simulink model "MVC2026_sim"  (R2023b)
settings: Solver=ode23t  StartTime=0.0  StopTime=inf  FixedStep=Ts  RelTol=1e-3
values from neighbouring files (symbols this model uses):
  saveDataSampling = 0.01    [main.m]
undefined symbols (not defined in the file or in its folder): BAT, BUS, CH, CTRLpmsm, DiscIntNeverNeededParam, EMS, LoadRef, MOT, TraceRef, Ts, VEH, WindRef
libraries: nesl_utility x50, fl_lib x28, ee_lib x19, simulink x9, slpidlib x5, eeTransforms x4, sdl_lib x4, batteryecm_lib x1, eeGeneralControl x1
(part 1 of 3)
settings Model: SimulationMode=accelerator  Creator=ortolud16324  LastModifiedBy=ortolud16324
settings SolverCC: SolverResetMethod=Robust
settings DebuggingCC: SignalRangeChecking=warning

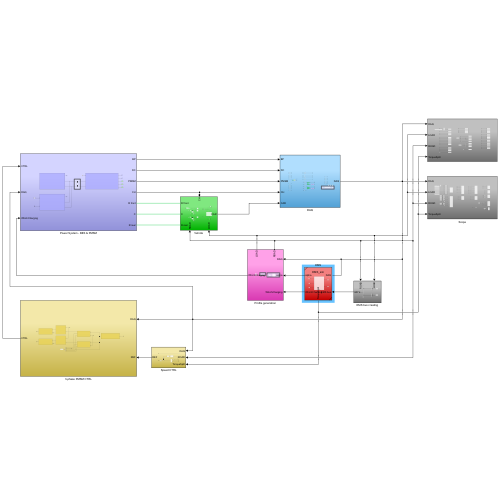
[thumbnail: Simulink's stored preview of the top-level diagram]
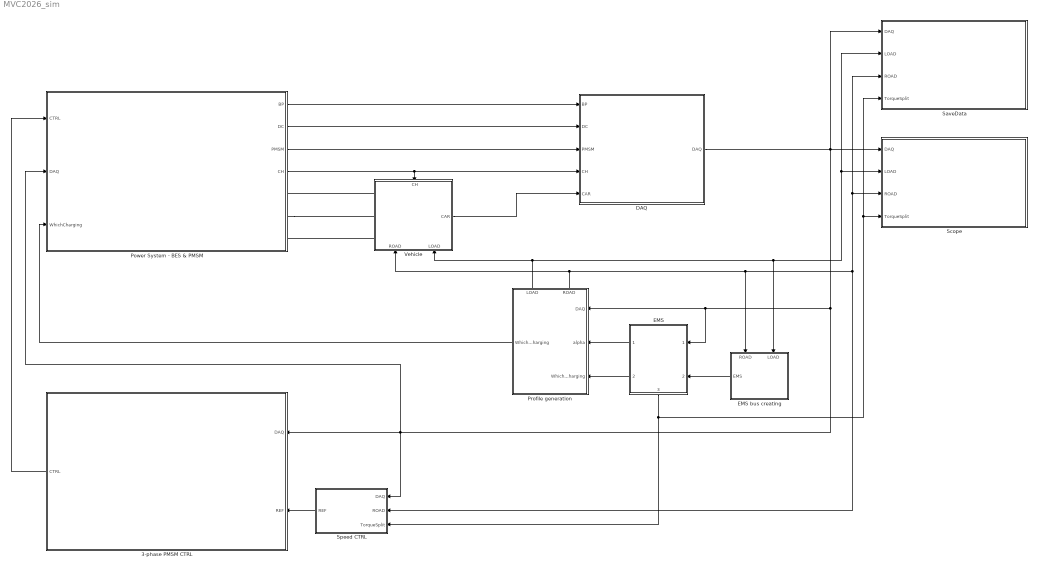
== system MVC2026_sim ==
  3-phase PMSM CTRL : Subsystem
  DAQ : Subsystem
  EMS : Subsystem  ReferencedSubsystem=EMS_sim
      settings: PortSchema="{\"entries\":[{\"content\":{\"sides\":[{\"content\":{\"connectorIds\":[\"In1\",\"In2\"]},\"type\":\"ConnectorPlacement.EquallySpacedRectSide\",\"uuid\":\"3854e963-bedd-46a1-9385-3ff6107fc6b9\"},{\"content\":{\"connectorIds\":[\"Out1\",\"Out2\"],\"side\":\"RIGHT\"},\"type\":\"ConnectorPlacement.EquallySpacedRectSide\",\"uuid\":\"f1426a81-f9cd-4ff1-8bf2-5f138fc7a080\"},{\"content\":{\"side\":\"TOP\"},\"type\":\"ConnectorPlacement.EquallySpacedRectSide\",\"uuid\":\"35da82e6-a4ef-4411-bef0-4d143ba62e69\"},{\"content\":{\"connectorIds\":[\"Out3\"],\"side\":\"BOTTOM\"},\"type\":\"ConnectorPlacement.EquallySpacedRectSide\",\"uuid\":\"49263484-0624-468a-bbdd-494b3d0a840d\"}]},\"type\":\"ConnectorPlacement.EquallySpacedConnector\",\"uuid\":\"bda56c1c-9437-4abe-9543-748b3b8cdce9\"}],\"packageUris\":[\"http://schema.mathworks.com/mf0/Connector/R2020b\"],\"version\":\"1.0\"}"
  EMS bus creating : Subsystem
      settings: PortSchema="{\"entries\":[{\"content\":{\"sides\":[{\"content\":{},\"type\":\"ConnectorPlacement.EquallySpacedRectSide\",\"uuid\":\"21c2c49d-f847-40d8-a3b7-36d147e58b7f\"},{\"content\":{\"connectorIds\":[\"Out1\"],\"side\":\"RIGHT\"},\"type\":\"ConnectorPlacement.EquallySpacedRectSide\",\"uuid\":\"241bf6a1-27e1-42c3-94c6-8bce09631f1d\"},{\"content\":{\"connectorIds\":[\"In1\",\"In2\"],\"side\":\"TOP\"},\"type\":\"ConnectorPlacement.EquallySpacedRectSide\",\"uuid\":\"b974af34-7c5b-4d4b-a896-f7169f3893eb\"}]},\"type\":\"ConnectorPlacement.EquallySpacedConnector\",\"uuid\":\"18f29ab8-c9e3-40d5-878b-a65cb8fef5da\"}],\"packageUris\":[\"http://schema.mathworks.com/mf0/Connector/R2020b\"],\"version\":\"1.0\"}"
  Power System - BES & PMSM : Subsystem
  Profile generation : Subsystem
      settings: PortSchema="{\"entries\":[{\"content\":{\"sides\":[{\"content\":{},\"type\":\"ConnectorPlacement.EquallySpacedRectSide\",\"uuid\":\"1924d7e1-ad70-4431-86e8-3c0ab7915ed9\"},{\"content\":{\"connectorIds\":[\"Out1\",\"Out2\"],\"side\":\"RIGHT\"},\"type\":\"ConnectorPlacement.EquallySpacedRectSide\",\"uuid\":\"609a06d3-9868-427b-9701-aec2c756f49e\"},{\"content\":{\"connectorIds\":[\"Out3\"],\"side\":\"TOP\"},\"type\":\"ConnectorPlacement.EquallySpacedRectSide\",\"uuid\":\"716e804f-913b-44a8-8dd3-1f544c7b7f23\"},{\"content\":{\"connectorIds\":[\"In1\",\"In2\",\"In3\"],\"side\":\"BOTTOM\"},\"type\":\"ConnectorPlacement.EquallySpacedRectSide\",\"uuid\":\"65f48948-cd5d-40ea-b4ca-71cadca582ae\"}]},\"type\":\"ConnectorPlacement.EquallySpacedConnector\",\"uuid\":\"7287addc-c47d-45e5-b586-b740e7da9654\"}],\"packageUris\":[\"http://schema.mathworks.com/mf0/Connector/R2020b\"],\"version\":\"1.0\"}"
  SaveData : Subsystem
  Scope : Subsystem
  Speed CTRL : Subsystem
  Vehicle : Subsystem
      settings: PortSchema="{\"entries\":[{\"content\":{\"sides\":[{\"content\":{\"connectorIds\":[\"LConn1\",\"LConn2\",\"LConn3\"]},\"type\":\"ConnectorPlacement.EquallySpacedRectSide\",\"uuid\":\"47b5f502-5a69-4856-a60d-9019b079dd3a\"},{\"content\":{\"connectorIds\":[\"Out1\"],\"side\":\"RIGHT\"},\"type\":\"ConnectorPlacement.EquallySpacedRectSide\",\"uuid\":\"3ad49b8f-ca2c-4bc9-b661-e3bc5c11dea5\"},{\"content\":{\"connectorIds\":[\"In1\"],\"side\":\"TOP\"},\"type\":\"ConnectorPlacement.EquallySpacedRectSide\",\"uuid\":\"b3b19f67-7f1f-4579-962f-8f7dd2f2f25f\"},{\"content\":{\"connectorIds\":[\"In2\",\"In3\"],\"side\":\"BOTTOM\"},\"type\":\"ConnectorPlacement.EquallySpacedRectSide\",\"uuid\":\"38380e36-a7be-41b3-b623-721420be15cb\"}]},\"type\":\"ConnectorPlacement.EquallySpacedConnector\",\"uuid\":\"551b2662-6f8a-4005-9043-ed2c26ef0cc2\"}],\"packageUris\":[\"http://schema.mathworks.com/mf0/Connector/R2020b\"],\"version\":\"1.0\"}"
  wires:
  Power System - BES & PMSM/1(BP) -> DAQ/1(BP)
  Power System - BES & PMSM/2(DC) -> DAQ/2(DC)
  Power System - BES & PMSM/3(PMSM) -> DAQ/3(PMSM)
  Power System - BES & PMSM/4(CH) -> DAQ/4(CH), Vehicle/1(CH)
  3-phase PMSM CTRL/1(CTRL) -> Power System - BES & PMSM/1(CTRL)
  Speed CTRL/1(REF) -> 3-phase PMSM CTRL/2(REF)
  Vehicle/1(CAR) -> DAQ/5(CAR)
  EMS bus creating/1(EMS) -> EMS/2
  DAQ/1(DAQ) -> Scope/1(DAQ), SaveData/1(DAQ), EMS/1, Profile generation/3(DAQ), Speed CTRL/1(DAQ), Power System - BES & PMSM/2(DAQ), 3-phase PMSM CTRL/1(DAQ)
  Profile generation/2(ROAD) -> SaveData/3(ROAD), Scope/3(ROAD), Speed CTRL/2(ROAD), EMS bus creating/2(ROAD), Vehicle/2(ROAD)
  Profile generation/1(LOAD) -> SaveData/2(LOAD), Scope/2(LOAD), EMS bus creating/1(LOAD), Vehicle/3(LOAD)
  Profile generation/3("WhichCharging ") -> Power System - BES & PMSM/3("WhichCharging ")
  EMS/3 -> Speed CTRL/3(TorqueSplit), Scope/4(TorqueSplit), SaveData/4(TorqueSplit)
  EMS/1 -> Profile generation/2(alpha)
  EMS/2 -> Profile generation/1(WhichCharging)
  connections:
  Vehicle/LConn1 -- Power System - BES & PMSM/RConn1
  Power System - BES & PMSM/RConn2 -- Vehicle/LConn2
  Vehicle/LConn3 -- Power System - BES & PMSM/RConn3

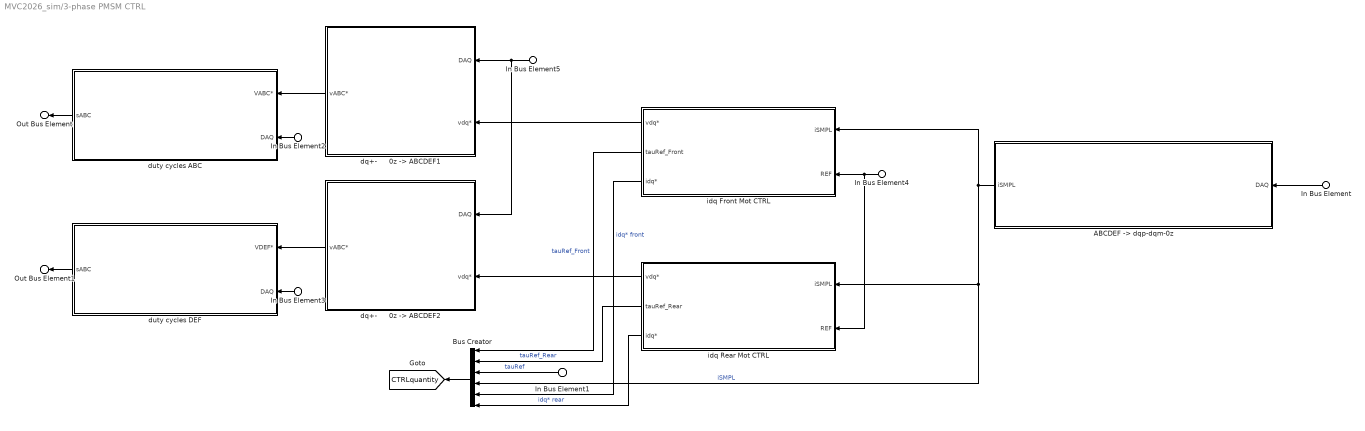
== system MVC2026_sim/3-phase PMSM CTRL ==
  In Bus Element{,2..3,5} (4 alike) : Inport  PortName=DAQ
  In Bus Element4 : Inport  Port=2  PortName=REF
  In Bus Element1 : Inport  Port=2  PortName=REF  Element=tau
  "ABCDEF -> dqp-dqm-0z" : Subsystem
  Bus Creator : BusCreator  Inputs=6
  "dq+-      0z -> ABCDEF1" : Subsystem
  "dq+-      0z -> ABCDEF2" : Subsystem
  duty cycles ABC : Subsystem
  duty cycles DEF : Subsystem
  idq Front Mot CTRL : Subsystem
  idq Rear Mot CTRL : Subsystem
  Out Bus Element : Outport  PortName=CTRL  Element=swFrontMot
  Out Bus Element1 : Outport  PortName=CTRL  Element=swRearMot
  tag scope: CTRLquantity=global
  wires:
  idq Front Mot CTRL/1(vdq*) -> "dq+-      0z -> ABCDEF1"/2(vdq*)
  duty cycles ABC/1(sABC) -> Out Bus Element/1
  In Bus Element/1 -> "ABCDEF -> dqp-dqm-0z"/1(DAQ)
  "dq+-      0z -> ABCDEF1"/1(vABC*) -> duty cycles ABC/1(VABC*)
  In Bus Element2/1 -> duty cycles ABC/2(DAQ)
  duty cycles DEF/1(sABC) -> Out Bus Element1/1
  In Bus Element3/1 -> duty cycles DEF/2(DAQ)
  idq Rear Mot CTRL/1(vdq*) -> "dq+-      0z -> ABCDEF2"/2(vdq*)
  In Bus Element4/1 -> idq Rear Mot CTRL/2(REF), idq Front Mot CTRL/2(REF)
  "dq+-      0z -> ABCDEF2"/1(vABC*) -> duty cycles DEF/1(VDEF*)
  "ABCDEF -> dqp-dqm-0z"/1(iSMPL) -> idq Rear Mot CTRL/1(iSMPL), Bus Creator/4, idq Front Mot CTRL/1(iSMPL)  "iSMPL"
  idq Front Mot CTRL/2(tauRef_Front) -> Bus Creator/1  "tauRef_Front"
  idq Rear Mot CTRL/2(tauRef_Rear) -> Bus Creator/2  "tauRef_Rear"
  In Bus Element1/1 -> Bus Creator/3  "tauRef"
  Bus Creator/1 -> [CTRLquantity]
  idq Front Mot CTRL/3(idq*) -> Bus Creator/5  "idq* front"
  idq Rear Mot CTRL/3(idq*) -> Bus Creator/6  "idq* rear"
  In Bus Element5/1 -> "dq+-      0z -> ABCDEF2"/1(DAQ), "dq+-      0z -> ABCDEF1"/1(DAQ)

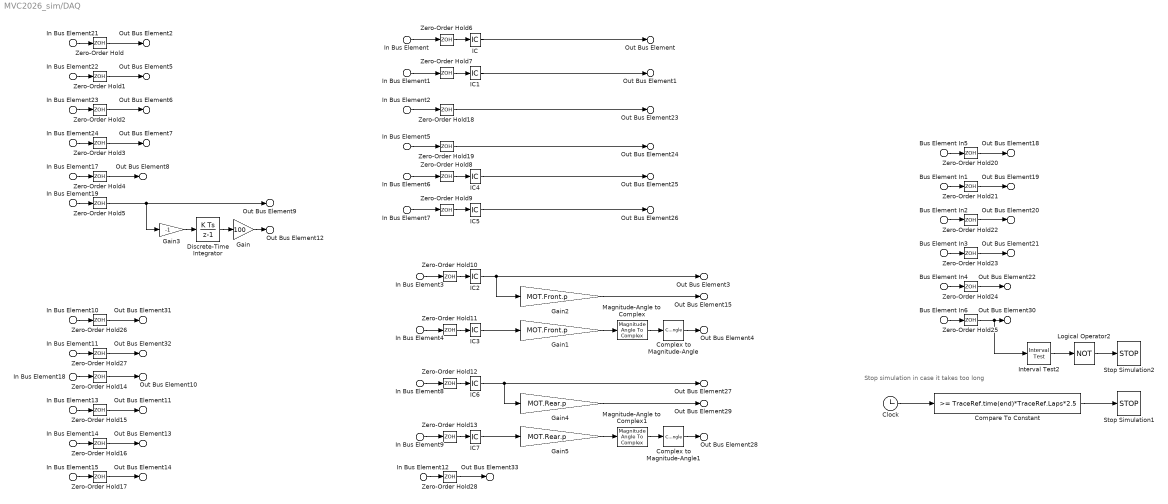
== system MVC2026_sim/DAQ ==
  note: Stop simulation in case it takes too long
  In Bus Element19 : Inport  PortName=BP  Element=iBP
  In Bus Element17 : Inport  PortName=BP  Element=vBP
  In Bus Element21 : Inport  Port=2  PortName=DC  Element=vFrontMot
  In Bus Element22 : Inport  Port=2  PortName=DC  Element=iFrontMot
  In Bus Element23 : Inport  Port=2  PortName=DC  Element=vRearMot
  In Bus Element24 : Inport  Port=2  PortName=DC  Element=iRearMot
  In Bus Element : Inport  Port=3  PortName=PMSM  Element=iFrontMot
  In Bus Element1 : Inport  Port=3  PortName=PMSM  Element=iRearMot
  In Bus Element3 : Inport  Port=3  PortName=PMSM  Element=wmFrontMot
  In Bus Element4 : Inport  Port=3  PortName=PMSM  Element=thmFrontMot
  In Bus Element5 : Inport  Port=3  PortName=PMSM  Element=TeFrontMot
  In Bus Element2 : Inport  Port=3  PortName=PMSM  Element=TeRearMot
  In Bus Element6 : Inport  Port=3  PortName=PMSM  Element=vFrontMot
  In Bus Element7 : Inport  Port=3  PortName=PMSM  Element=vRearMot
  In Bus Element8 : Inport  Port=3  PortName=PMSM  Element=wmRearMot
  In Bus Element9 : Inport  Port=3  PortName=PMSM  Element=thmRearMot
  In Bus Element18 : Inport  Port=4  PortName=CH  Element=vPLUG
  In Bus Element13 : Inport  Port=4  PortName=CH  Element=iPLUG
  In Bus Element14 : Inport  Port=4  PortName=CH  Element=vWPT
  In Bus Element15 : Inport  Port=4  PortName=CH  Element=iWPT
  In Bus Element10 : Inport  Port=4  PortName=CH  Element=vEMERGENCY
  In Bus Element11 : Inport  Port=4  PortName=CH  Element=iEMERGENCY
  In Bus Element12 : Inport  Port=4  PortName=CH  Element=Braking
  Bus Element In5 : Inport  Port=5  PortName=CAR  Element=Speed
  Bus Element In1 : Inport  Port=5  PortName=CAR  Element=VerForceFront
  Bus Element In2 : Inport  Port=5  PortName=CAR  Element=VerForceRear
  Bus Element In3 : Inport  Port=5  PortName=CAR  Element=wmFrTyre
  Bus Element In4 : Inport  Port=5  PortName=CAR  Element=wmReTyre
  Bus Element In6 : Inport  Port=5  PortName=CAR  Element=Position
  Clock : Clock
  Compare To Constant : simulink/Logic and Bit Operations/Compare To Constant  relop=>=  const=TraceRef.time(end)*TraceRef.Laps*2.5  OutDataTypeStr=boolean
  Complex to Magnitude-Angle : ComplexToMagnitudeAngle  Output=Angle
  Complex to Magnitude-Angle1 : ComplexToMagnitudeAngle  Output=Angle
  Discrete-Time Integrator : DiscreteIntegrator  gainval=1/BAT.Q_nom  InitialCondition=BAT.SoC_0  SampleTime=Ts  ICPrevOutput=DiscIntNeverNeededParam  ICPrevScaledInput=DiscIntNeverNeededParam
  Gain : Gain  Gain=100
  Gain1 : Gain  Gain=MOT.Front.p
  Gain2 : Gain  Gain=MOT.Front.p
  Gain3 : Gain  Gain=-1
  Gain4 : Gain  Gain=MOT.Rear.p
  Gain5 : Gain  Gain=MOT.Rear.p
  IC{,1..7} (8 alike) : InitialCondition  Value=0
  Interval Test2 : simulink/Logic and Bit Operations/Interval Test  IntervalClosedRight=on  uplimit=TraceRef.Laps * TraceRef.PosRef(end)  IntervalClosedLeft=on  lowlimit=-TraceRef.Laps * TraceRef.PosRef(end)  OutDataTypeStr=boolean
  Logical Operator2 : Logic  Operator=NOT  AllPortsSameDT=off  OutDataTypeStr=boolean
  Magnitude-Angle to Complex : MagnitudeAngleToComplex  Input=Angle  ConstantPart=1
  Magnitude-Angle to Complex1 : MagnitudeAngleToComplex  Input=Angle  ConstantPart=1
  Stop Simulation1 : Stop
  Stop Simulation2 : Stop
  Zero-Order Hold{,1..28} (29 alike) : ZeroOrderHold  SampleTime=Ts
  Out Bus Element : Outport  PortName=DAQ  Element=iFrontMot
  Out Bus Element1 : Outport  PortName=DAQ  Element=iRearMot
  Out Bus Element2 : Outport  PortName=DAQ  Element=vDCFrontMot
  Out Bus Element3 : Outport  PortName=DAQ  Element=wmFrontMotor
  Out Bus Element4 : Outport  PortName=DAQ  Element=thmeFrontMotor
  Out Bus Element5 : Outport  PortName=DAQ  Element=iDCFrontMot
  Out Bus Element6 : Outport  PortName=DAQ  Element=vDCRearMot
  Out Bus Element7 : Outport  PortName=DAQ  Element=iDCRearMot
  Out Bus Element8 : Outport  PortName=DAQ  Element=vBP
  Out Bus Element9 : Outport  PortName=DAQ  Element=iBP
  Out Bus Element12 : Outport  PortName=DAQ  Element=SoC_BP
  Out Bus Element15 : Outport  PortName=DAQ  Element=wmeFrontMotor
  Out Bus Element10 : Outport  PortName=DAQ  Element=vPLUG
  Out Bus Element11 : Outport  PortName=DAQ  Element=iPLUG
  Out Bus Element13 : Outport  PortName=DAQ  Element=vWPT
  Out Bus Element14 : Outport  PortName=DAQ  Element=iWPT
  Out Bus Element18 : Outport  PortName=DAQ  Element=CarSpeed
  Out Bus Element19 : Outport  PortName=DAQ  Element=VerForceFront
  Out Bus Element20 : Outport  PortName=DAQ  Element=VerForceRear
  Out Bus Element21 : Outport  PortName=DAQ  Element=wmFrTyre
  Out Bus Element22 : Outport  PortName=DAQ  Element=wmReTyre
  Out Bus Element23 : Outport  PortName=DAQ  Element=TeRearMot
  Out Bus Element24 : Outport  PortName=DAQ  Element=TeFrontMot
  Out Bus Element25 : Outport  PortName=DAQ  Element=vFrontMot
  Out Bus Element26 : Outport  PortName=DAQ  Element=vRearMot
  Out Bus Element27 : Outport  PortName=DAQ  Element=wmRearMotor
  Out Bus Element28 : Outport  PortName=DAQ  Element=thmeRearMotor
  Out Bus Element29 : Outport  PortName=DAQ  Element=wmeRearMotor
  Out Bus Element30 : Outport  PortName=DAQ  Element=Position
  Out Bus Element31 : Outport  PortName=DAQ  Element=vEMERGENCY
  Out Bus Element32 : Outport  PortName=DAQ  Element=iEMERGENCY
  Out Bus Element33 : Outport  PortName=DAQ  Element=Braking
  wires:
  Discrete-Time Integrator/1 -> Gain/1
  Zero-Order Hold7/1 -> IC1/1
  Zero-Order Hold11/1 -> IC3/1
  Zero-Order Hold10/1 -> IC2/1
  Zero-Order Hold/1 -> Out Bus Element2/1
  Gain3/1 -> Discrete-Time Integrator/1
  In Bus Element19/1 -> Zero-Order Hold5/1
  Zero-Order Hold5/1 -> Out Bus Element9/1, Gain3/1
  Zero-Order Hold4/1 -> Out Bus Element8/1
  In Bus Element17/1 -> Zero-Order Hold4/1
  Zero-Order Hold2/1 -> Out Bus Element6/1
  In Bus Element24/1 -> Zero-Order Hold3/1
  Zero-Order Hold3/1 -> Out Bus Element7/1
  In Bus Element22/1 -> Zero-Order Hold1/1
  Zero-Order Hold1/1 -> Out Bus Element5/1
  In Bus Element5/1 -> Zero-Order Hold19/1
  In Bus Element3/1 -> Zero-Order Hold10/1
  In Bus Element1/1 -> Zero-Order Hold7/1
  In Bus Element/1 -> Zero-Order Hold6/1
  Magnitude-Angle to Complex/1 -> Complex to Magnitude-Angle/1
  Complex to Magnitude-Angle/1 -> Out Bus Element4/1
  Gain1/1 -> Magnitude-Angle to Complex/1
  IC3/1 -> Gain1/1
  In Bus Element4/1 -> Zero-Order Hold11/1
  IC2/1 -> Out Bus Element3/1, Gain2/1
  IC1/1 -> Out Bus Element1/1
  IC/1 -> Out Bus Element/1
  Zero-Order Hold15/1 -> Out Bus Element11/1
  Zero-Order Hold17/1 -> Out Bus Element14/1
  Zero-Order Hold16/1 -> Out Bus Element13/1
  Zero-Order Hold14/1 -> Out Bus Element10/1
  In Bus Element18/1 -> Zero-Order Hold14/1
  In Bus Element13/1 -> Zero-Order Hold15/1
  In Bus Element14/1 -> Zero-Order Hold16/1
  In Bus Element15/1 -> Zero-Order Hold17/1
  In Bus Element2/1 -> Zero-Order Hold18/1
  Zero-Order Hold20/1 -> Out Bus Element18/1
  Zero-Order Hold24/1 -> Out Bus Element22/1
  Zero-Order Hold22/1 -> Out Bus Element20/1
  Zero-Order Hold23/1 -> Out Bus Element21/1
  Zero-Order Hold21/1 -> Out Bus Element19/1
  Bus Element In4/1 -> Zero-Order Hold24/1
  Bus Element In3/1 -> Zero-Order Hold23/1
  Bus Element In2/1 -> Zero-Order Hold22/1
  Bus Element In1/1 -> Zero-Order Hold21/1
  Bus Element In5/1 -> Zero-Order Hold20/1
  Zero-Order Hold18/1 -> Out Bus Element23/1
  Zero-Order Hold19/1 -> Out Bus Element24/1
  IC5/1 -> Out Bus Element26/1
  Zero-Order Hold8/1 -> IC4/1
  Zero-Order Hold9/1 -> IC5/1
  IC6/1 -> Gain4/1, Out Bus Element27/1
  In Bus Element9/1 -> Zero-Order Hold13/1
  IC7/1 -> Gain5/1
  Gain5/1 -> Magnitude-Angle to Complex1/1
  Complex to Magnitude-Angle1/1 -> Out Bus Element28/1
  Magnitude-Angle to Complex1/1 -> Complex to Magnitude-Angle1/1
  In Bus Element8/1 -> Zero-Order Hold12/1
  Zero-Order Hold12/1 -> IC6/1
  Zero-Order Hold13/1 -> IC7/1
  Gain/1 -> Out Bus Element12/1
  Bus Element In6/1 -> Zero-Order Hold25/1
  Logical Operator2/1 -> Stop Simulation2/1
  Interval Test2/1 -> Logical Operator2/1
  Zero-Order Hold25/1 -> Interval Test2/1, Out Bus Element30/1
  In Bus Element21/1 -> Zero-Order Hold/1
  In Bus Element23/1 -> Zero-Order Hold2/1
  In Bus Element6/1 -> Zero-Order Hold8/1
  In Bus Element7/1 -> Zero-Order Hold9/1
  Zero-Order Hold6/1 -> IC/1
  Gain2/1 -> Out Bus Element15/1
  Gain4/1 -> Out Bus Element29/1
  In Bus Element11/1 -> Zero-Order Hold27/1
  In Bus Element10/1 -> Zero-Order Hold26/1
  Zero-Order Hold26/1 -> Out Bus Element31/1
  Zero-Order Hold27/1 -> Out Bus Element32/1
  In Bus Element12/1 -> Zero-Order Hold28/1
  Zero-Order Hold28/1 -> Out Bus Element33/1
  IC4/1 -> Out Bus Element25/1
  Clock/1 -> Compare To Constant/1
  Compare To Constant/1 -> Stop Simulation1/1

== system MVC2026_sim/EMS bus creating ==
  LOAD : Inport
  ROAD : Inport  Port=2
  Bus Creator1 : BusCreator  Inputs=2
  Bus Selector : BusSelector  OutputSignals=speedProfile  OutputAsBus=on
  Bus Selector1 : BusSelector  OutputSignals=Mass  OutputAsBus=on
  EMS : Outport
  wires:
  ROAD/1 -> Bus Selector/1
  LOAD/1 -> Bus Selector1/1
  Bus Selector/1 -> Bus Creator1/1  "speedProfile"
  Bus Selector1/1 -> Bus Creator1/2  "Mass"
  Bus Creator1/1 -> EMS/1

== system MVC2026_sim/Power System - BES & PMSM ==
  note: Refrigeration
  In Bus Element : Inport  PortName=CTRL
  Bus Element In3 : Inport  Port=2  PortName=DAQ
  "WhichCharging " : Inport  Port=3
  Battery : Subsystem
  Charging system : Subsystem
  PMSMs drive : Subsystem
  Resistor : fl_lib/Electrical/Electrical Elements/Resistor  R=400 Ohm  i_specify=off  i_priority=None  i=0 A  i_nominal_specify=off  i_nominal_unit=A  i_nominal_value=1  v_specify=off  v_priority=None  v=0 V  v_nominal_specify=off  v_nominal_unit=V  v_nominal_value=1
  R front : PMIOPort  Side=Right
  C : PMIOPort  Port=2  Side=Right
  R rear : PMIOPort  Port=3  Side=Right
  Out Bus Element2 : Outport  PortName=BP
  Out Bus Element14 : Outport  Port=2  PortName=DC
  Out Bus Element1 : Outport  Port=3  PortName=PMSM
  Out Bus Element3 : Outport  Port=4  PortName=CH
  wires:
  PMSMs drive/1(DC) -> Out Bus Element14/1
  Battery/1(BP) -> Out Bus Element2/1
  In Bus Element/1 -> PMSMs drive/1(CTRL)
  PMSMs drive/2(PMSM) -> Out Bus Element1/1
  Charging system/1(CH) -> Out Bus Element3/1
  "WhichCharging "/1 -> Charging system/1(WhichCharging)
  Bus Element In3/1 -> Charging system/2(DAQ)
  connections:
  Battery/RConn2 -- Charging system/RConn2 -- Resistor/RConn1 -- PMSMs drive/LConn2
  R front/RConn1 -- PMSMs drive/RConn1
  C/RConn1 -- PMSMs drive/RConn2
  R rear/RConn1 -- PMSMs drive/RConn3
  Battery/RConn1 -- Charging system/RConn1 -- Resistor/LConn1 -- PMSMs drive/LConn1

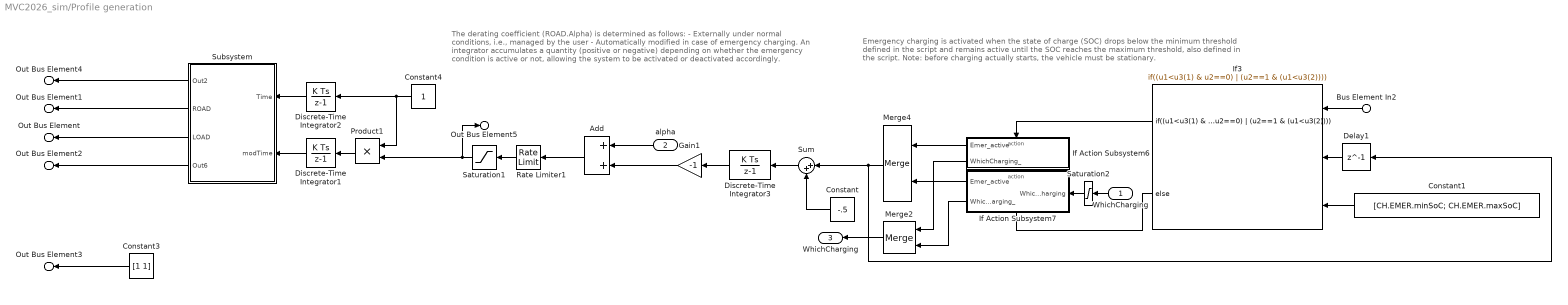
== system MVC2026_sim/Profile generation ==
  note: Emergency charging is activated when the state of charge (SOC) drops below the minimum threshold defined in the script and remains active until the SOC
      | reaches the maximum threshold, also defined in the script.
      | Note: before charging actually starts, the vehicle must be stationary.
  note: The derating coefficient (ROAD.Alpha) is determined as follows:
      | - Externally under normal conditions, i.e., managed by the user
      | - Automatically modified in case of emergency charging.
      | An integrator accumulates a quantity (positive or negative) depending on
      | whether the emergency condition is active or not,
      | allowing the system to be activated or deactivated accordingly.
  WhichCharging : Inport
  alpha : Inport  Port=2
  Bus Element In2 : Inport  Port=3  PortName=DAQ  Element=SoC_BP
  Add : Sum
  Constant : Constant  Value=-.5  SampleTime=Ts
  Constant1 : Constant  Value=[CH.EMER.minSoC; CH.EMER.maxSoC]
  Constant3 : Constant  Value=[1 1]  SampleTime=Ts
  Constant4 : Constant  SampleTime=Ts
  Delay1 : Delay  DelayLength=1
  Discrete-Time Integrator1 : DiscreteIntegrator  SampleTime=Ts  ICPrevOutput=DiscIntNeverNeededParam  ICPrevScaledInput=DiscIntNeverNeededParam
  Discrete-Time Integrator2 : DiscreteIntegrator  SampleTime=Ts  ICPrevOutput=DiscIntNeverNeededParam  ICPrevScaledInput=DiscIntNeverNeededParam
  Discrete-Time Integrator3 : DiscreteIntegrator  SampleTime=Ts  LimitOutput=on  UpperSaturationLimit=1  LowerSaturationLimit=0  ICPrevOutput=DiscIntNeverNeededParam  ICPrevScaledInput=DiscIntNeverNeededParam
  Gain1 : Gain  Gain=-1
  If Action Subsystem6 : Subsystem  TreatAsAtomicUnit=on
  If Action Subsystem7 : Subsystem  TreatAsAtomicUnit=on
  If3 : If  NumInputs=3  IfExpression=(u1<u3(1) & u2==0) | (u2==1 & (u1<u3(2)))
  Merge2 : Merge
  Merge4 : Merge
  Product1 : Product
  Rate Limiter1 : RateLimiter  RisingSlewLimit=0.5  FallingSlewLimit=-0.15  SampleTimeMode=inherited  InitialCondition=1
  Saturation1 : Saturate  UpperLimit=1  LowerLimit=0
  Saturation2 : Saturate  UpperLimit=2  LowerLimit=0
  Subsystem : Subsystem
  Sum : Sum  Inputs=|++
  Out Bus Element : Outport  PortName=LOAD  Element=Mass
  Out Bus Element3 : Outport  PortName=LOAD  Element=CG
  Out Bus Element1 : Outport  Port=2  PortName=ROAD  Element=windSpeed
  Out Bus Element2 : Outport  Port=2  PortName=ROAD  Element=angle
  Out Bus Element4 : Outport  Port=2  PortName=ROAD  Element=speedProfile
  Out Bus Element5 : Outport  Port=2  PortName=ROAD  Element=Alpha
  "WhichCharging " : Outport  Port=3
  wires:
  Constant3/1 -> Out Bus Element3/1
  Constant4/1 -> Discrete-Time Integrator2/1, Product1/1
  Discrete-Time Integrator1/1 -> Subsystem/2(modTime)
  Product1/1 -> Discrete-Time Integrator1/1
  Saturation1/1 -> Out Bus Element5/1, Product1/2
  Discrete-Time Integrator2/1 -> Subsystem/1(Time)
  Subsystem/1(Out2) -> Out Bus Element4/1
  Rate Limiter1/1 -> Saturation1/1
  If Action Subsystem6/1(Emer_active) -> Merge4/1
  If Action Subsystem7/1(Emer_active) -> Merge4/2
  Delay1/1 -> If3/2
  If3/2 -> If Action Subsystem7/Action
  Bus Element In2/1 -> If3/1
  If3/1 -> If Action Subsystem6/Action
  Merge4/1 -> Delay1/1, Sum/1
  Add/1 -> Rate Limiter1/1
  Discrete-Time Integrator3/1 -> Gain1/1
  Gain1/1 -> Add/2
  Constant/1 -> Sum/2
  Sum/1 -> Discrete-Time Integrator3/1
  Constant1/1 -> If3/3
  WhichCharging/1 -> Saturation2/1
  If Action Subsystem6/2(WhichCharging_) -> Merge2/1
  If Action Subsystem7/2(WhichCharging_) -> Merge2/2
  Merge2/1 -> "WhichCharging "/1
  alpha/1 -> Add/1
  Saturation2/1 -> If Action Subsystem7/1(WhichCharging)
  Subsystem/4(Out6) -> Out Bus Element2/1
  Subsystem/3(LOAD) -> Out Bus Element/1
  Subsystem/2(ROAD) -> Out Bus Element1/1

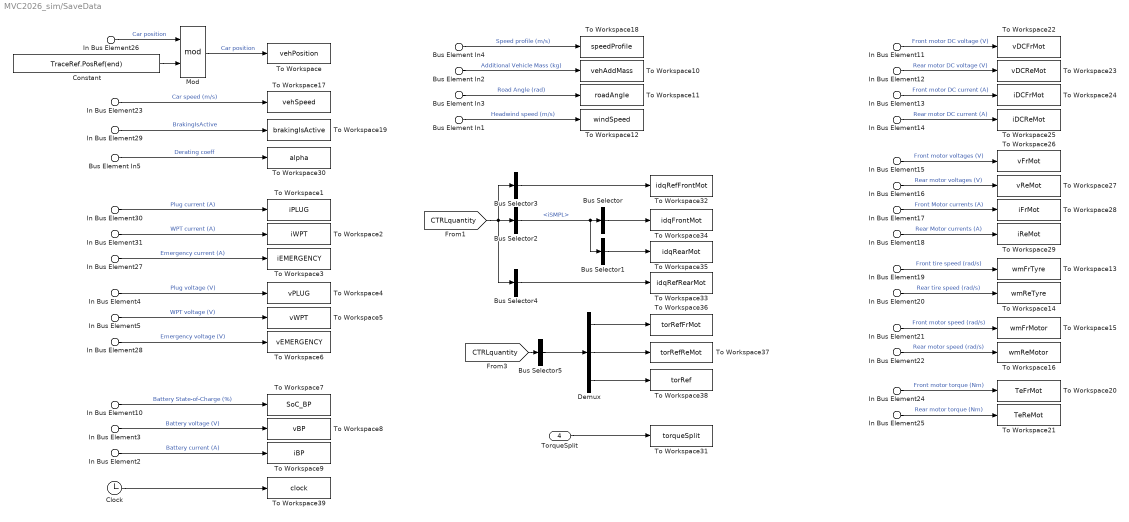
== system MVC2026_sim/SaveData ==
  In Bus Element10 : Inport  PortName=DAQ  Element=SoC_BP
  In Bus Element2 : Inport  PortName=DAQ  Element=iBP
  In Bus Element3 : Inport  PortName=DAQ  Element=vBP
  In Bus Element4 : Inport  PortName=DAQ  Element=vPLUG
  In Bus Element5 : Inport  PortName=DAQ  Element=vWPT
  In Bus Element30 : Inport  PortName=DAQ  Element=iPLUG
  In Bus Element31 : Inport  PortName=DAQ  Element=iWPT
  In Bus Element14 : Inport  PortName=DAQ  Element=iDCRearMot
  In Bus Element17 : Inport  PortName=DAQ  Element=iFrontMot
  In Bus Element15 : Inport  PortName=DAQ  Element=vFrontMot
  In Bus Element16 : Inport  PortName=DAQ  Element=vRearMot
  In Bus Element18 : Inport  PortName=DAQ  Element=iRearMot
  In Bus Element11 : Inport  PortName=DAQ  Element=vDCFrontMot
  In Bus Element12 : Inport  PortName=DAQ  Element=vDCRearMot
  In Bus Element13 : Inport  PortName=DAQ  Element=iDCFrontMot
  In Bus Element19 : Inport  PortName=DAQ  Element=wmFrTyre
  In Bus Element20 : Inport  PortName=DAQ  Element=wmReTyre
  In Bus Element21 : Inport  PortName=DAQ  Element=wmFrontMotor
  In Bus Element22 : Inport  PortName=DAQ  Element=wmRearMotor
  In Bus Element23 : Inport  PortName=DAQ  Element=CarSpeed
  In Bus Element24 : Inport  PortName=DAQ  Element=TeFrontMot
  In Bus Element25 : Inport  PortName=DAQ  Element=TeRearMot
  In Bus Element26 : Inport  PortName=DAQ  Element=Position
  In Bus Element27 : Inport  PortName=DAQ  Element=iEMERGENCY
  In Bus Element28 : Inport  PortName=DAQ  Element=vEMERGENCY
  In Bus Element29 : Inport  PortName=DAQ  Element=Braking
  Bus Element In2 : Inport  Port=2  PortName=LOAD  Element=Mass
  Bus Element In3 : Inport  Port=3  PortName=ROAD  Element=angle
  Bus Element In1 : Inport  Port=3  PortName=ROAD  Element=windSpeed
  Bus Element In4 : Inport  Port=3  PortName=ROAD  Element=speedProfile
  Bus Element In5 : Inport  Port=3  PortName=ROAD  Element=Alpha
  TorqueSplit : Inport  Port=4
  Bus Selector : BusSelector  OutputSignals=idq0FrontMotor  OutputAsBus=on
  Bus Selector1 : BusSelector  OutputSignals=idq0RearMotor  OutputAsBus=on
  Bus Selector2 : BusSelector  OutputSignals=iSMPL
  Bus Selector3 : BusSelector  OutputSignals=idq* front  OutputAsBus=on
  Bus Selector4 : BusSelector  OutputSignals=idq* rear  OutputAsBus=on
  Bus Selector5 : BusSelector  OutputSignals=tauRef_Front,tauRef_Rear,tauRef  OutputAsBus=on
  Clock : Clock
  Constant : Constant  Value=TraceRef.PosRef(end)  SampleTime=Inf
  Demux : Demux  Outputs=3
  Mod : Math  Operator=mod
  To Workspace : ToWorkspace  VariableName=vehPosition  SaveFormat=Timeseries  SampleTime=saveDataSampling
  To Workspace1 : ToWorkspace  VariableName=iPLUG  SaveFormat=Timeseries  SampleTime=saveDataSampling
  To Workspace10 : ToWorkspace  VariableName=vehAddMass  SaveFormat=Timeseries  SampleTime=saveDataSampling
  To Workspace11 : ToWorkspace  VariableName=roadAngle  SaveFormat=Timeseries  SampleTime=saveDataSampling
  To Workspace12 : ToWorkspace  VariableName=windSpeed  SaveFormat=Timeseries  SampleTime=saveDataSampling
  To Workspace13 : ToWorkspace  VariableName=wmFrTyre  SaveFormat=Timeseries  SampleTime=saveDataSampling
  To Workspace14 : ToWorkspace  VariableName=wmReTyre  SaveFormat=Timeseries  SampleTime=saveDataSampling
  To Workspace15 : ToWorkspace  VariableName=wmFrMotor  SaveFormat=Timeseries  SampleTime=saveDataSampling
  To Workspace16 : ToWorkspace  VariableName=wmReMotor  SaveFormat=Timeseries  SampleTime=saveDataSampling
  To Workspace17 : ToWorkspace  VariableName=vehSpeed  SaveFormat=Timeseries  SampleTime=saveDataSampling
  To Workspace18 : ToWorkspace  VariableName=speedProfile  SaveFormat=Timeseries  SampleTime=saveDataSampling
  To Workspace19 : ToWorkspace  VariableName=brakingIsActive  SaveFormat=Timeseries  SampleTime=saveDataSampling
  To Workspace2 : ToWorkspace  VariableName=iWPT  SaveFormat=Timeseries  SampleTime=saveDataSampling
  To Workspace20 : ToWorkspace  VariableName=TeFrMot  SaveFormat=Timeseries  SampleTime=saveDataSampling
  To Workspace21 : ToWorkspace  VariableName=TeReMot  SaveFormat=Timeseries  SampleTime=saveDataSampling
  To Workspace22 : ToWorkspace  VariableName=vDCFrMot  SaveFormat=Timeseries  SampleTime=saveDataSampling
  To Workspace23 : ToWorkspace  VariableName=vDCReMot  SaveFormat=Timeseries  SampleTime=saveDataSampling
  To Workspace24 : ToWorkspace  VariableName=iDCFrMot  SaveFormat=Timeseries  SampleTime=saveDataSampling
  To Workspace25 : ToWorkspace  VariableName=iDCReMot  SaveFormat=Timeseries  SampleTime=saveDataSampling
  To Workspace26 : ToWorkspace  VariableName=vFrMot  SaveFormat=Timeseries  SampleTime=saveDataSampling
  To Workspace27 : ToWorkspace  VariableName=vReMot  SaveFormat=Timeseries  SampleTime=saveDataSampling
  To Workspace28 : ToWorkspace  VariableName=iFrMot  SaveFormat=Timeseries  SampleTime=saveDataSampling
  To Workspace29 : ToWorkspace  VariableName=iReMot  SaveFormat=Timeseries  SampleTime=saveDataSampling
  To Workspace3 : ToWorkspace  VariableName=iEMERGENCY  SaveFormat=Timeseries  SampleTime=saveDataSampling
  To Workspace30 : ToWorkspace  VariableName=alpha  SaveFormat=Timeseries  SampleTime=saveDataSampling
  To Workspace31 : ToWorkspace  VariableName=torqueSplit  SaveFormat=Timeseries  SampleTime=saveDataSampling
  To Workspace32 : ToWorkspace  VariableName=idqRefFrontMot  SaveFormat=Timeseries  SampleTime=saveDataSampling
  To Workspace33 : ToWorkspace  VariableName=idqRefRearMot  SaveFormat=Timeseries  SampleTime=saveDataSampling
  To Workspace34 : ToWorkspace  VariableName=idqFrontMot  SaveFormat=Timeseries  SampleTime=saveDataSampling
  To Workspace35 : ToWorkspace  VariableName=idqRearMot  SaveFormat=Timeseries  SampleTime=saveDataSampling
  To Workspace36 : ToWorkspace  VariableName=torRefFrMot  SaveFormat=Timeseries  SampleTime=saveDataSampling
  To Workspace37 : ToWorkspace  VariableName=torRefReMot  SaveFormat=Timeseries  SampleTime=saveDataSampling
  To Workspace38 : ToWorkspace  VariableName=torRef  SaveFormat=Timeseries  SampleTime=saveDataSampling
  To Workspace39 : ToWorkspace  VariableName=clock  SaveFormat=Timeseries  SampleTime=saveDataSampling
  To Workspace4 : ToWorkspace  VariableName=vPLUG  SaveFormat=Timeseries  SampleTime=saveDataSampling
  To Workspace5 : ToWorkspace  VariableName=vWPT  SaveFormat=Timeseries  SampleTime=saveDataSampling
  To Workspace6 : ToWorkspace  VariableName=vEMERGENCY  SaveFormat=Timeseries  SampleTime=saveDataSampling
  To Workspace7 : ToWorkspace  VariableName=SoC_BP  SaveFormat=Timeseries  SampleTime=saveDataSampling
  To Workspace8 : ToWorkspace  VariableName=vBP  SaveFormat=Timeseries  SampleTime=saveDataSampling
  To Workspace9 : ToWorkspace  VariableName=iBP  SaveFormat=Timeseries  SampleTime=saveDataSampling
  wires:
  Bus Element In2/1 -> To Workspace10/1  "Additional Vehicle Mass (kg)"
  Bus Element In3/1 -> To Workspace11/1  "Road Angle (rad)"
  Bus Element In1/1 -> To Workspace12/1  "Headwind speed (m/s)"
  In Bus Element3/1 -> To Workspace8/1  "Battery voltage (V)"
  In Bus Element2/1 -> To Workspace9/1  "Battery current (A)"
  In Bus Element4/1 -> To Workspace4/1  "Plug voltage (V)"
  In Bus Element5/1 -> To Workspace5/1  "WPT voltage (V)"
  In Bus Element10/1 -> To Workspace7/1  "Battery State-of-Charge (%)"
  In Bus Element15/1 -> To Workspace26/1  "Front motor voltages (V)"
  In Bus Element16/1 -> To Workspace27/1  "Rear motor voltages (V)"
  In Bus Element17/1 -> To Workspace28/1  "Front Motor currents (A)"
  In Bus Element18/1 -> To Workspace29/1  "Rear Motor currents (A)"
  In Bus Element11/1 -> To Workspace22/1  "Front motor DC voltage (V)"
  In Bus Element12/1 -> To Workspace23/1  "Rear motor DC voltage (V)"
  In Bus Element13/1 -> To Workspace24/1  "Front motor DC current (A)"
  In Bus Element14/1 -> To Workspace25/1  "Rear motor DC current (A)"
  In Bus Element19/1 -> To Workspace13/1  "Front tire speed (rad/s)"
  In Bus Element20/1 -> To Workspace14/1  "Rear tire speed (rad/s)"
  In Bus Element21/1 -> To Workspace15/1  "Front motor speed (rad/s)"
  In Bus Element22/1 -> To Workspace16/1  "Rear motor speed (rad/s)"
  In Bus Element25/1 -> To Workspace21/1  "Rear motor torque (Nm)"
  In Bus Element24/1 -> To Workspace20/1  "Front motor torque (Nm)"
  In Bus Element23/1 -> To Workspace17/1  "Car speed (m/s)"
  Bus Element In4/1 -> To Workspace18/1  "Speed profile (m/s)"
  In Bus Element26/1 -> Mod/1  "Car position"
  Bus Selector/1 -> To Workspace34/1
  Bus Selector3/1 -> To Workspace32/1
  In Bus Element27/1 -> To Workspace3/1  "Emergency current (A)"
  In Bus Element28/1 -> To Workspace6/1  "Emergency voltage (V)"
  Constant/1 -> Mod/2
  In Bus Element29/1 -> To Workspace19/1  "BrakingIsActive"
  Bus Element In5/1 -> To Workspace30/1  "Derating coeff"
  In Bus Element30/1 -> To Workspace1/1  "Plug current (A)"
  In Bus Element31/1 -> To Workspace2/1  "WPT current (A)"
  Bus Selector2/1 -> Bus Selector/1, Bus Selector1/1  "<iSMPL>"
  [CTRLquantity] -> Bus Selector4/1, Bus Selector3/1, Bus Selector2/1
  Bus Selector4/1 -> To Workspace33/1
  [CTRLquantity] -> Bus Selector5/1
  Bus Selector5/1 -> Demux/1
  TorqueSplit/1 -> To Workspace31/1
  Mod/1 -> To Workspace/1  "Car position"
  Bus Selector1/1 -> To Workspace35/1
  Demux/1 -> To Workspace36/1
  Demux/2 -> To Workspace37/1
  Demux/3 -> To Workspace38/1
  Clock/1 -> To Workspace39/1

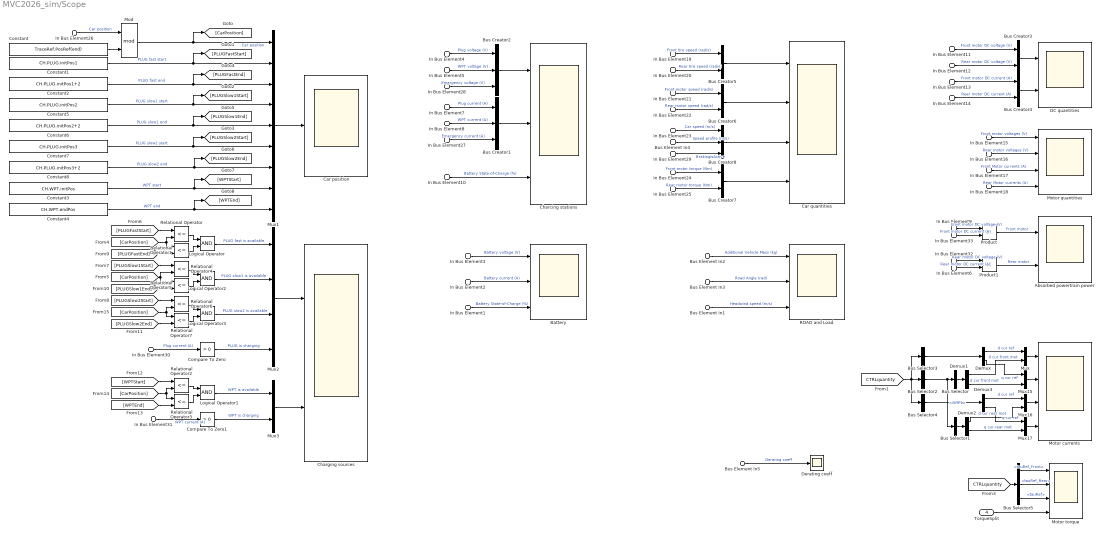
== system MVC2026_sim/Scope ==
  In Bus Element1 : Inport  PortName=DAQ  Element=SoC_BP
  In Bus Element10 : Inport  PortName=DAQ  Element=SoC_BP
  In Bus Element2 : Inport  PortName=DAQ  Element=iBP
  In Bus Element3 : Inport  PortName=DAQ  Element=vBP
  In Bus Element4 : Inport  PortName=DAQ  Element=vPLUG
  In Bus Element5 : Inport  PortName=DAQ  Element=vWPT
  In Bus Element7 : Inport  PortName=DAQ  Element=iPLUG
  In Bus Element30 : Inport  PortName=DAQ  Element=iPLUG
  In Bus Element8 : Inport  PortName=DAQ  Element=iWPT
  In Bus Element31 : Inport  PortName=DAQ  Element=iWPT
  In Bus Element14 : Inport  PortName=DAQ  Element=iDCRearMot
  In Bus Element6 : Inport  PortName=DAQ  Element=iDCRearMot
  In Bus Element17 : Inport  PortName=DAQ  Element=iFrontMot
  In Bus Element15 : Inport  PortName=DAQ  Element=vFrontMot
  In Bus Element16 : Inport  PortName=DAQ  Element=vRearMot
  In Bus Element18 : Inport  PortName=DAQ  Element=iRearMot
  In Bus Element11 : Inport  PortName=DAQ  Element=vDCFrontMot
  In Bus Element9 : Inport  PortName=DAQ  Element=vDCFrontMot
  In Bus Element12 : Inport  PortName=DAQ  Element=vDCRearMot
  In Bus Element32 : Inport  PortName=DAQ  Element=vDCRearMot
  In Bus Element13 : Inport  PortName=DAQ  Element=iDCFrontMot
  In Bus Element33 : Inport  PortName=DAQ  Element=iDCFrontMot
  In Bus Element19 : Inport  PortName=DAQ  Element=wmFrTyre
  In Bus Element20 : Inport  PortName=DAQ  Element=wmReTyre
  In Bus Element21 : Inport  PortName=DAQ  Element=wmFrontMotor
  In Bus Element22 : Inport  PortName=DAQ  Element=wmRearMotor
  In Bus Element23 : Inport  PortName=DAQ  Element=CarSpeed
  In Bus Element24 : Inport  PortName=DAQ  Element=TeFrontMot
  In Bus Element25 : Inport  PortName=DAQ  Element=TeRearMot
  In Bus Element26 : Inport  PortName=DAQ  Element=Position
  In Bus Element27 : Inport  PortName=DAQ  Element=iEMERGENCY
  In Bus Element28 : Inport  PortName=DAQ  Element=vEMERGENCY
  In Bus Element29 : Inport  PortName=DAQ  Element=Braking
  Bus Element In2 : Inport  Port=2  PortName=LOAD  Element=Mass
  Bus Element In3 : Inport  Port=3  PortName=ROAD  Element=angle
  Bus Element In1 : Inport  Port=3  PortName=ROAD  Element=windSpeed
  Bus Element In4 : Inport  Port=3  PortName=ROAD  Element=speedProfile
  Bus Element In5 : Inport  Port=3  PortName=ROAD  Element=Alpha
  TorqueSplit : Inport  Port=4
  Absorbed powertrain power : Scope  NumInputPorts=2
  Battery : Scope  NumInputPorts=3
  Bus Creator1 : BusCreator  Inputs=3
  Bus Creator2 : BusCreator  Inputs=3
  Bus Creator{3..7} (5 alike) : BusCreator  Inputs=2
  Bus Creator8 : BusCreator  Inputs=3
  Bus Selector : BusSelector  OutputSignals=idq0FrontMotor  OutputAsBus=on
  Bus Selector1 : BusSelector  OutputSignals=idq0RearMotor  OutputAsBus=on
  Bus Selector2 : BusSelector  OutputSignals=iSMPL
  Bus Selector3 : BusSelector  OutputSignals=idq* front  OutputAsBus=on
  Bus Selector4 : BusSelector  OutputSignals=idq* rear  OutputAsBus=on
  Bus Selector5 : BusSelector  OutputSignals=tauRef_Front,tauRef_Rear,tauRef
  Car position : Scope
  Car quantities : Scope  NumInputPorts=4
  Charcing stations : Scope  NumInputPorts=3
  Charging sources : Scope  NumInputPorts=2
  Compare To Zero : simulink/Logic and Bit Operations/Compare To Zero  relop=>  OutDataTypeStr=boolean
  Compare To Zero1 : simulink/Logic and Bit Operations/Compare To Zero  relop=>  OutDataTypeStr=boolean
  Constant : Constant  Value=TraceRef.PosRef(end)
  Constant1 : Constant  Value=CH.PLUG.initPos1
  Constant2 : Constant  Value=CH.PLUG.initPos1+2
  Constant3 : Constant  Value=CH.WPT.initPos
  Constant4 : Constant  Value=CH.WPT.endPos
  Constant5 : Constant  Value=CH.PLUG.initPos2
  Constant6 : Constant  Value=CH.PLUG.initPos2+2
  Constant7 : Constant  Value=CH.PLUG.initPos3
  Constant8 : Constant  Value=CH.PLUG.initPos3+2
  DC quantities : Scope  NumInputPorts=2
  Demux{,1..3} (4 alike) : Demux  Outputs=2
  Derating coeff : Scope
  Logical Operator{,1..3} (4 alike) : Logic  AllPortsSameDT=off  OutDataTypeStr=boolean
  Mod : Math  Operator=mod
  Motor currents : Scope  NumInputPorts=4
  Motor quantities : Scope  NumInputPorts=4
  Motor torque : Scope  NumInputPorts=4
  Mux{,3,15..17} (5 alike) : Mux  Inputs=2
  Mux1 : Mux  Inputs=9
  Mux2 : Mux
  Product : Product
  Product1 : Product
  ROAD and Load : Scope  NumInputPorts=3
  Relational Operator{,1..7} (8 alike) : RelationalOperator  Operator=<=  OutDataTypeStr=boolean  RndMeth=Simplest  InputSameDT=off
  wires:
  Bus Element In2/1 -> ROAD and Load/1  "Additional Vehicle Mass (kg)"
  Bus Element In3/1 -> ROAD and Load/2  "Road Angle (rad)"
  Bus Element In1/1 -> ROAD and Load/3  "Headwind speed (m/s)"
  In Bus Element3/1 -> Battery/1  "Battery voltage (V)"
  In Bus Element2/1 -> Battery/2  "Battery current (A)"
  In Bus Element1/1 -> Battery/3  "Battery State-of-Charge (%)"
  Bus Creator2/1 -> Charcing stations/1
  Bus Creator1/1 -> Charcing stations/2
  In Bus Element7/1 -> Bus Creator1/1  "Plug current (A)"
  In Bus Element4/1 -> Bus Creator2/1  "Plug voltage (V)"
  In Bus Element5/1 -> Bus Creator2/2  "WPT voltage (V)"
  In Bus Element8/1 -> Bus Creator1/2  "WPT current (A)"
  In Bus Element10/1 -> Charcing stations/3  "Battery State-of-Charge (%)"
  In Bus Element15/1 -> Motor quantities/1  "Front motor voltages (V)"
  In Bus Element16/1 -> Motor quantities/2  "Rear motor voltages (V)"
  In Bus Element17/1 -> Motor quantities/3  "Front Motor currents (A)"
  In Bus Element18/1 -> Motor quantities/4  "Rear Motor currents (A)"
  In Bus Element11/1 -> Bus Creator3/1  "Front motor DC voltage (V)"
  In Bus Element12/1 -> Bus Creator3/2  "Rear motor DC voltage (V)"
  In Bus Element13/1 -> Bus Creator4/1  "Front motor DC current (A)"
  In Bus Element14/1 -> Bus Creator4/2  "Rear motor DC current (A)"
  Bus Creator3/1 -> DC quantities/1
  Bus Creator4/1 -> DC quantities/2
  In Bus Element19/1 -> Bus Creator5/1  "Front tire speed (rad/s)"
  In Bus Element20/1 -> Bus Creator5/2  "Rear tire speed (rad/s)"
  In Bus Element21/1 -> Bus Creator6/1  "Front motor speed (rad/s)"
  In Bus Element22/1 -> Bus Creator6/2  "Rear motor speed (rad/s)"
  In Bus Element25/1 -> Bus Creator7/2  "Rear motor torque (Nm)"
  In Bus Element24/1 -> Bus Creator7/1  "Front motor torque (Nm)"
  Bus Creator5/1 -> Car quantities/1
  Bus Creator6/1 -> Car quantities/2
  Bus Creator7/1 -> Car quantities/4
  Bus Creator8/1 -> Car quantities/3
  In Bus Element23/1 -> Bus Creator8/1  "Car speed (m/s)"
  Bus Element In4/1 -> Bus Creator8/2  "Speed profile (m/s)"
  In Bus Element26/1 -> Mod/1  "Car position"
  Demux/1 -> Mux/1  "d cur ref"
  Mux15/1 -> Motor currents/2
  Mux/1 -> Motor currents/1
  Mux16/1 -> Motor currents/3
  Mux17/1 -> Motor currents/4
  Demux/2 -> Mux15/1  "q cur ref"
  Bus Selector/1 -> Demux1/1
  Demux1/1 -> Mux/2  "d cur front mot"
  Demux1/2 -> Mux15/2  "d cur front mot"
  Demux2/2 -> Mux17/2  "q cur rear mot"
  Demux2/1 -> Mux16/2  "d cur rear mot"
  Bus Selector1/1 -> Demux2/1
  Bus Selector3/1 -> Demux/1
  In Bus Element27/1 -> Bus Creator1/3  "Emergency current (A)"
  In Bus Element28/1 -> Bus Creator2/3  "Emergency voltage (V)"
  Constant/1 -> Mod/2
  In Bus Element29/1 -> Bus Creator8/3  "BrakingIsActive"
  Bus Element In5/1 -> Derating coeff/1  "Derating coeff"
  Mux1/1 -> Car position/1
  Constant1/1 -> [PLUGFastStart], Mux1/2  "PLUG fast start"
  Constant2/1 -> [PLUGFastEnd], Mux1/3  "PLUG fast end"
  Relational Operator/1 -> Logical Operator/1
  Relational Operator1/1 -> Logical Operator/2
  In Bus Element30/1 -> Compare To Zero/1  "Plug current (A)"
  Mux2/1 -> Charging sources/1
  Logical Operator/1 -> Mux2/1  "PLUG fast is available"
  Compare To Zero/1 -> Mux2/4  "PLUG is charging"
  Compare To Zero1/1 -> Mux3/2  "WPT is charging"
  Logical Operator1/1 -> Mux3/1  "WPT is available"
  Mux3/1 -> Charging sources/2
  In Bus Element31/1 -> Compare To Zero1/1  "WPT current (A)"
  Relational Operator3/1 -> Logical Operator1/2
  Relational Operator2/1 -> Logical Operator1/1
  Constant4/1 -> [WPTEnd], Mux1/9  "WPT end"
  Constant3/1 -> [WPTStart], Mux1/8  "WPT start"
  Product/1 -> Absorbed powertrain power/1  "Front motor"
  Product1/1 -> Absorbed powertrain power/2  "Rear motor"
  In Bus Element6/1 -> Product1/2  "Rear motor DC current (A)"
  In Bus Element33/1 -> Product/2  "Front motor DC current (A)"
  In Bus Element32/1 -> Product1/1  "Rear motor DC voltage (V)"
  In Bus Element9/1 -> Product/1  "Front motor DC voltage (V)"
  Bus Selector2/1 -> Bus Selector/1, Bus Selector1/1  "<iSMPL>"
  [CTRLquantity] -> Bus Selector4/1, Bus Selector3/1, Bus Selector2/1
  Bus Selector4/1 -> Demux3/1
  Demux3/1 -> Mux16/1  "d cur ref"
  Demux3/2 -> Mux17/1  "q cur ref"
  [CTRLquantity] -> Bus Selector5/1
  Bus Selector5/1 -> Motor torque/1  "<tauRef_Front>"
  TorqueSplit/1 -> Motor torque/4
  Constant5/1 -> [PLUGSlow1Start], Mux1/4  "PLUG slow1 start"
  Constant6/1 -> [PLUGSlow1End], Mux1/5  "PLUG slow1 end"
  Constant7/1 -> Mux1/6, [PLUGSlow2Start]  "PLUG slow2 start"
  Constant8/1 -> [PLUGSlow2End], Mux1/7  "PLUG slow2 end"
  Logical Operator2/1 -> Mux2/2  "PLUG slow1 is available"
  Relational Operator5/1 -> Logical Operator2/2
  Relational Operator4/1 -> Logical Operator2/1
  Relational Operator6/1 -> Logical Operator3/1
  Relational Operator7/1 -> Logical Operator3/2
  Logical Operator3/1 -> Mux2/3  "PLUG slow2 is available"
  Mod/1 -> [CarPosition], Mux1/1  "Car position"
  [CarPosition] -> Relational Operator/2, Relational Operator1/1
  [CarPosition] -> Relational Operator4/2, Relational Operator5/1
  [PLUGFastStart] -> Relational Operator/1
  [PLUGSlow1Start] -> Relational Operator4/1
  [PLUGSlow2Start] -> Relational Operator6/1
  [PLUGFastEnd] -> Relational Operator1/2
  [PLUGSlow1End] -> Relational Operator5/2
  [PLUGSlow2End] -> Relational Operator7/2
  [WPTStart] -> Relational Operator2/1
  [WPTEnd] -> Relational Operator3/2
  [CarPosition] -> Relational Operator3/1, Relational Operator2/2
  [CarPosition] -> Relational Operator6/2, Relational Operator7/1
  Bus Selector5/2 -> Motor torque/2  "<tauRef_Rear>"
  Bus Selector5/3 -> Motor torque/3  "<tauRef>"

== system MVC2026_sim/Speed CTRL ==
  In Bus Element : Inport  PortName=DAQ  Element=CarSpeed
  In Bus Element2 : Inport  PortName=DAQ  Element=Braking
  In Bus Element1 : Inport  Port=2  PortName=ROAD  Element=speedProfile
  TorqueSplit : Inport  Port=3
  Discrete Derivative : simulink/Quick Insert/Discrete/Discrete Derivative  gainval=1.0  ICPrevScaledInput=0.0  OutMin=[]  OutMax=[]  OutDataType=fixdt(1, 16)  OutScaling=2^-10  DoSatur=off
  Gain : Gain  Gain=0.05*(MOT.Front.Tenom + MOT.Rear.Tenom)
  Low-Pass Filter (Discrete or Continuous) : eeGeneralControl/Low-Pass Filter (Discrete or Continuous)  K=1  T=1/(2*pi*5)  B=inf  A=-inf  init_option=Inherited from block input  x0=0  Ts=Ts
  PID Controller : slpidlib/PID Controller  Controller=PI  Form=Parallel  TimeDomain=Discrete-time  UseExternalTs=off  SampleTime=Ts  IntegratorMethod=Forward Euler  FilterMethod=Forward Euler  ControllerParametersSource=internal  P=61.8429493344261  I=30.126734069317  UseKiTs=off  D=0  N=100  UseFilter=on  TunerSelectOption=Transfer Function Based (PID Tuner App)  InitialConditionSource=internal  InitialConditionForIntegrator=0  InitialConditionForFilter=0  DifferentiatorICPrevScaledInput=0  ExternalReset=level  TrackingMode=off  Kt=1  LimitOutput=on  SatLimitsSource=internal  UpperSaturationLimit=MOT.Front.Tenom + MOT.Rear.Tenom  LowerSaturationLimit=-(MOT.Front.Tenom + MOT.Rear.Tenom)  LinearizeAsGain=on  AntiWindupMode=clamping  Kb=1  LimitIntegrator=off  UpperIntegratorSaturationLimit=MOT.Front.Tenom + MOT.Rear.Tenom  LowerIntegratorSaturationLimit=-(MOT.Front.Tenom + MOT.Rear.Tenom)  POutMin=[]  POutMax=[]  IOutMin=[]  IOutMax=[]  DOutMin=[]  DOutMax=[]  NOutMin=[]  NOutMax=[]  SumOutMin=[]  SumOutMax=[]  SaturationOutMin=[]  SaturationOutMax=[]  PParamMin=[]  PParamMax=[]  IParamMin=[]  IParamMax=[]  DParamMin=[]  DParamMax=[]  NParamMin=[]  NParamMax=[]  KbParamMin=[]  KbParamMax=[]  KtParamMin=[]  KtParamMax=[]  KbOutMin=[]  KbOutMax=[]  KtOutMin=[]  KtOutMax=[]  IntegratorOutMin=[]  IntegratorOutMax=[]  FilterOutMin=[]  FilterOutMax=[]  SumI1OutMin=[]  SumI1OutMax=[]  SumI2OutMin=[]  SumI2OutMax=[]  SumI3OutMin=[]  SumI3OutMax=[]  SumI4OutMin=[]  SumI4OutMax=[]  SumDOutMin=[]  SumDOutMax=[]  DifferentiatorOutMin=[]  DifferentiatorOutMax=[]  FilterDiffOutCoefMin=[]  FilterDiffOutCoefMax=[]  ReciprocalOutMin=[]  ReciprocalOutMax=[]  SumDenOutMin=[]  SumDenOutMax=[]  SumNumOutMin=[]  SumNumOutMax=[]  DivideOutMin=[]  DivideOutMax=[]  UdiffTsProdOutMin=[]  UdiffTsProdOutMax=[]  NTsProdOutMin=[]  NTsProdOutMax=[]  UintegralTsProdOutMin=[]  UintegralTsProdOutMax=[]  UngainTsProdOutMin=[]  UngainTsProdOutMax=[]  ClampingZeroOutDataTypeStr=Inherit: Inherit via back propagation  ClampingZeroOutMin=[]  ClampingZeroOutMax=[]  FilterDenConstantOutDataTypeStr=Inherit: Inherit via back propagation  FilterDenConstantOutMin=[]  FilterDenConstantOutMax=[]  PCopyOutDataTypeStr=Inherit: Inherit via back propagation  PCopyOutMin=[]  PCopyOutMax=[]  NCopyOutDataTypeStr=Inherit: Inherit via back propagation  NCopyOutMin=[]  NCopyOutMax=[]  IntegratorContinuousStateAttributes=''  IntegratorStateMustResolveToSignalObject=off  IntegratorRTWStateStorageClass=Auto  FilterContinuousStateAttributes=''  FilterStateMustResolveToSignalObject=off  FilterRTWStateStorageClass=Auto  ParallelPVariant=InternalParameters  IdealPVariant=Disabled  IVariant=InternalParameters  DVariant=Disabled  IntegratorVariant=Discrete  SatVariant=Enabled  AWVariant=DiscClampingParallel  PCopyVariant=Disabled  TRVariant=Disabled  FdbkBlocksVariant=Forward  IdealPFdbkVariant=Disabled  SatFdbkVariant=Disabled  DerivativeFilterVariant=Disabled  NVariant=Disabled  NCopyVariant=Disabled_SignalSpec  FilterICVariant=Disabled  IntegratorICVariant=InternalICs  ExternalResetVariant=ExternalReset  TRSumVariant=Passthrough  SumFdbkVariant=Disabled  SumVariant=Sum_PI  TsampFilterVariant=InternalTs  TsampNgainVariant=Passthrough  TsampIntegralVariant=Disabled_SignalSpec  ExternalSaturationOutDataTypeStr=Inherit: Same as second input
  Saturation : Saturate  UpperLimit=MOT.Front.Tenom + MOT.Rear.Tenom  LowerLimit=-(MOT.Front.Tenom + MOT.Rear.Tenom)
  Sum : Sum  Inputs=|+-
  Sum1 : Sum  Inputs=++|
  Out Bus Element : Outport  PortName=REF  Element=tau
  Out Bus Element1 : Outport  PortName=REF  Element=torquesplit
  wires:
  Sum/1 -> PID Controller/1
  In Bus Element/1 -> Sum/2
  In Bus Element1/1 -> Low-Pass Filter (Discrete or Continuous)/1, Sum/1
  In Bus Element2/1 -> PID Controller/2
  TorqueSplit/1 -> Out Bus Element1/1
  PID Controller/1 -> Sum1/2
  Sum1/1 -> Saturation/1
  Saturation/1 -> Out Bus Element/1
  Low-Pass Filter (Discrete or Continuous)/1 -> Discrete Derivative/1
  Discrete Derivative/1 -> Gain/1
  Gain/1 -> Sum1/1
